simulink model "CSE_Lab3_No1_ReducedBlockDiagram_Simulink"  (R2023b)
settings: Solver=VariableStepAuto  StartTime=0.0  StopTime=20  RelTol=1e-3
values from neighbouring files (symbols this model uses):
  TF_den = conv(TF4_den,TF6_den)    [CSE_Lab3_No1_ReducedBlockDiagram.m]
  TF_num = conv(TF4_num,TF6_num)    [CSE_Lab3_No1_ReducedBlockDiagram.m]
settings Model: Creator=Sofia Katrina Dilag  LastModifiedBy=Sofia Katrina Dilag

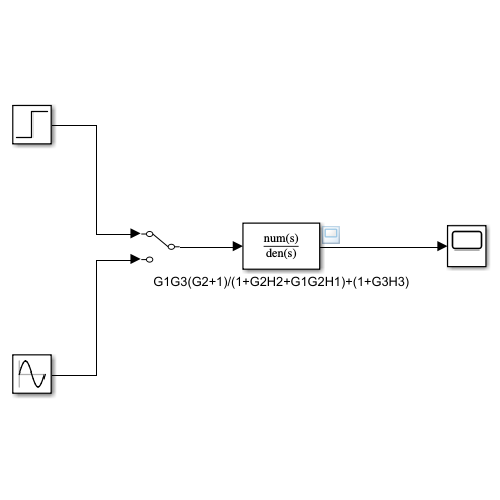
[thumbnail: Simulink's stored preview of the top-level diagram]
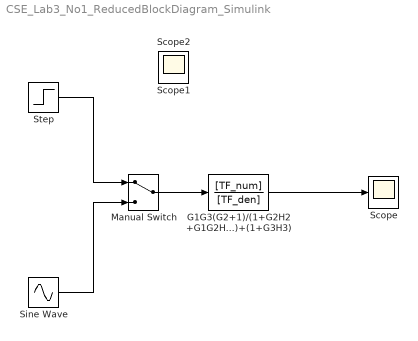
== system CSE_Lab3_No1_ReducedBlockDiagram_Simulink ==
  G1G3(G2+1)/(1+G2H2+G1G2H1)+(1+G3H3) : TransferFcn  Numerator=[TF_num]  Denominator=[TF_den]
  Manual Switch : ManualSwitch
  Scope : Scope
  Sine Wave : Sin  SampleTime=0
  Step : Step  Time=0  Before=0.1  SampleTime=0
  Scope1 : Scope
  Scope2 : Scope
  wires:
  G1G3(G2+1)/(1+G2H2+G1G2H1)+(1+G3H3)/1 -> Scope/1
  Step/1 -> Manual Switch/1
  Sine Wave/1 -> Manual Switch/2
  Manual Switch/1 -> G1G3(G2+1)/(1+G2H2+G1G2H1)+(1+G3H3)/1
